simulink model "Z_3Dctrl"  (R2023a)
settings: Solver=ode1  StartTime=0.0  StopTime=inf  FixedStep=0.001  RelTol=1e-3  EnableMultiTasking=on
PostLoadFcn:
  | , if any(exist('dsrtsu_mdlpostloadfcn', 'file') ~= 0), dsrtsu_mdlpostloadfcn('Execute', bdroot); end,
InitFcn:
  | , if any(exist('rtifpga_mdlclblib', 'file') ~= 0), rtifpga_mdlclblib('Init', bdroot); end,
  | [b,a] = butter(6,0.6)
  | z0_default = 0.080001
  | fatness_default = 1
  | offset_default = 0
  | scale_default = 0
  | tic
model workspace (MAT data in the model file):
  Iters = 5
  N_coils = 6
  fatness_default = 1
  running = 0
  z0_default = 0.080001
undefined symbols (not defined in the file or in its folder): a, b, DiscIntNeverNeededParam
libraries: dspstat3 x7, simulink x5, commfilt2 x3, rti2004lib x3, rtilibm x1
(part 2 of 3)

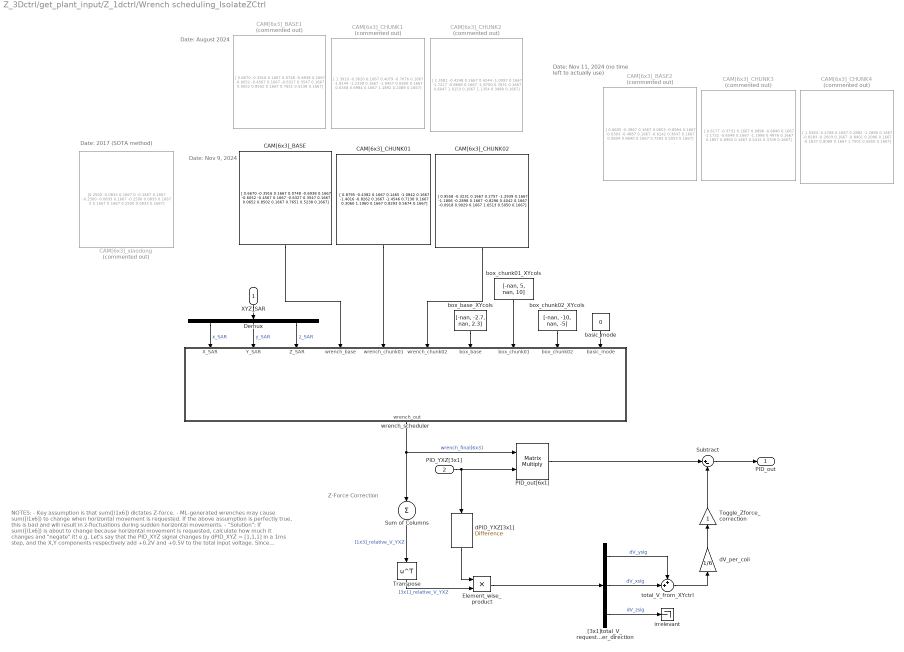
== system Z_3Dctrl/get_plant_input/Z_1dctrl/Wrench scheduling_IsolateZCtrl ==
  note: Date: August 2024
  note: Z-Force Correction
  note: NOTES:
      | - Key assumption is that sum([i1x6]) dictates Z-force.
      | - ML-generated wrenches may cause sum([i1x6]) to change when horizontal movement is requested. If the above assumption is perfectly true, this is bad and will result in z-fluctuations during sudden horizontal movements.
      | - "Solution": If sum([i1x6]) is about to change because horizontal movement is requested, calculate how much it changes and "negate" it!
      |
      | e.g. Let's say that the PID_XYZ signal changes by dPID_XYZ = [1,1,1] in a 1ms step, and the X,Y components respectively add +0.2V and +0.5V to the total input voltage.
      | Since sum(v[1x6]) is about to be +0.7V larger from horizontal motions alone (which is BAD since the sum, responsible for z-force, should be unaffected by horizontal motions), we "negate" this effect by subtracting (0.7V / 6 coils) = 0.11667V from EACH COIL in the final v[1x6] signal !
  note: Date: Nov 9, 2024
  note: Date: Nov 11, 2024
      | (no time left to actually use)
  note: Date: 2017 (SOTA method)
  XYZ_SAR : Inport
  PID_YXZ[3x1] : Inport  Port=2
  CAM[6x3]_BASE : Constant  Value=|
      | [    0.6670    -0.3916    0.1667
      |     0.0748    -0.6938    0.1667
      |    -0.6052   -0.4567    0.1667
      |    -0.6327   0.3547    0.1667
      |     0.0652   0.8502    0.1667
      |     0.7651   0.5238    0.1667]
  CAM[6x3]_BASE1 : Constant  Commented=on  Value=|
      | [    0.6670    -0.3916    0.1667
      |     0.0748    -0.6938    0.1667
      |    -0.6052   -0.4567    0.1667
      |    -0.6327   0.3547    0.1667
      |     0.0652   0.8502    0.1667
      |     0.7651   0.5238    0.1667]
  CAM[6x3]_BASE2 : Constant  Commented=on  Value=|
      | [    0.6605   -0.3967    0.1667
      |     0.0653   -0.8994    0.1667
      |    -0.6303   -0.4887    0.1667
      |    -0.6242    0.3647    0.1667
      |     0.0604    0.8640    0.1667
      |     0.7583    0.5053    0.1667]
  CAM[6x3]_CHUNK01 : Constant  Value=|
      | [    0.8795   -0.4382    0.1667
      |     0.1465   -1.0842    0.1667
      |    -1.4016   -0.8262    0.1667
      |    -1.4546    0.7130    0.1667
      |     0.3060    1.1960    0.1667
      |     0.8293    0.5674    0.1667]
  CAM[6x3]_CHUNK02 : Constant  Value=|
      | [   0.9558   -0.3231    0.1667
      |     0.2757   -1.2939    0.1667
      |    -1.1806   -0.2898    0.1667
      |    -0.8296    0.4042    0.1667
      |    -0.0918    0.9029    0.1667
      |     1.6513    0.5050    0.1667]
  CAM[6x3]_CHUNK1 : Constant  Commented=on  Value=|
      | [    1.3910    -0.3620    0.1667
      |     0.4079    -0.7676    0.1667
      |    -1.8144    -1.2338    0.1667
      |    -1.9457   0.6900    0.1667
      |     0.6358   0.6984    0.1667
      |     1.1892   0.2089    0.1667]
  CAM[6x3]_CHUNK2 : Constant  Commented=on  Value=|
      | [    1.3581    -0.4248    0.1667
      |     0.4244    -1.0097    0.1667
      |    -1.7217    -0.8668    0.1667
      |    -1.8700   0.7631    0.1667
      |     0.6047   1.0153    0.1667
      |     1.1354   0.3480    0.1667]
  CAM[6x3]_CHUNK3 : Constant  Commented=on  Value=|
      | [      0.6177   -0.3731    0.1667
      |     0.0896   -0.6840    0.1667
      |    -1.1732   -0.6548    0.1667
      |    -1.1996    0.4976    0.1667
      |     0.1857    0.6983    0.1667
      |     0.5415    0.3709    0.1667]
  CAM[6x3]_CHUNK4 : Constant  Commented=on  Value=|
      | [     1.0384   -0.4768    0.1667
      |     0.2882   -1.2890    0.1667
      |    -0.8283   -0.2003    0.1667
      |    -0.8401    0.2096    0.1667
      |    -0.1837    0.8089    0.1667
      |     1.7501    0.5650    0.1667]
  CAM[6x3]_xiaodong : Constant  Commented=on  Value=|
      | [0.2500    -0.0833    0.1667
      |          0    -0.1667    0.1667
      |    -0.2500    -0.0833    0.1667
      |    -0.2500   0.0833    0.1667
      |          0   0.1667    0.1667
      |     0.2500   0.0833    0.1667]
  Demux : Demux  Outputs=3
  Element_wise_product : Product
  PID_out[6x1] : Product  Multiplication=Matrix(*)
  Subtract : Sum  Inputs=|+-
  Sum of Columns : Sum  Inputs=+  CollapseMode=Specified dimension
  Toggle_Zforce_correction : Gain
  Transpose : Math  Operator=transpose
  "[3x1]total_V_requested_per_direction" : Demux  Outputs=3
  basic_mode : Constant  Value=0
  box_base_XYcols : Constant  Value=|
      | [-nan, -2.7,
      | nan, 2.3]
  box_chunk01_XYcols : Constant  Value=|
      | [-nan, 5,
      | nan, 10]
  box_chunk02_XYcols : Constant  Value=|
      | [-nan, -10,
      | nan, -5]
  dPID_YXZ[3x1] : simulink/Discrete/Difference  ICPrevInput=0.0  OutMin=[]  OutMax=[]  OutDataType=fixdt(1, 16)  OutScaling=2^-10  DoSatur=off
  dV_per_coil : Gain  Gain=1/6
  irrelevant : Terminator
  total_V_from_XYctrl : Sum  Inputs=++|
  wrench_scheduler : MATLAB Function  TreatAsAtomicUnit=on
  PID_out : Outport
  wires:
  CAM[6x3]_CHUNK02/1 -> wrench_scheduler/6(wrench_chunk02)
  box_chunk01_XYcols/1 -> wrench_scheduler/8(box_chunk01)
  basic_mode/1 -> wrench_scheduler/10(basic_mode)
  CAM[6x3]_BASE/1 -> wrench_scheduler/4(wrench_base)
  XYZ_SAR/1 -> Demux/1
  wrench_scheduler/1(wrench_out) -> Sum of Columns/1, PID_out[6x1]/1  "wrench_final[6x3]"
  Demux/3 -> wrench_scheduler/3(Z_SAR)  "z_SAR"
  box_base_XYcols/1 -> wrench_scheduler/7(box_base)
  CAM[6x3]_CHUNK01/1 -> wrench_scheduler/5(wrench_chunk01)
  Demux/2 -> wrench_scheduler/2(Y_SAR)  "y_SAR"
  Demux/1 -> wrench_scheduler/1(X_SAR)  "x_SAR"
  box_chunk02_XYcols/1 -> wrench_scheduler/9(box_chunk02)
  PID_out[6x1]/1 -> Subtract/1
  Sum of Columns/1 -> Transpose/1  "[1x3]_relative_V_YXZ"
  "[3x1]total_V_requested_per_direction"/1 -> total_V_from_XYctrl/1  "dV_ysig"
  "[3x1]total_V_requested_per_direction"/2 -> total_V_from_XYctrl/2  "dV_xsig"
  "[3x1]total_V_requested_per_direction"/3 -> irrelevant/1  "dV_zsig"
  PID_YXZ[3x1]/1 -> PID_out[6x1]/2, dPID_YXZ[3x1]/1
  Transpose/1 -> Element_wise_product/2  "[3x1]_relative_V_YXZ"
  Element_wise_product/1 -> "[3x1]total_V_requested_per_direction"/1
  dPID_YXZ[3x1]/1 -> Element_wise_product/1
  total_V_from_XYctrl/1 -> dV_per_coil/1
  dV_per_coil/1 -> Toggle_Zforce_correction/1
  Subtract/1 -> PID_out/1
  Toggle_Zforce_correction/1 -> Subtract/2

== system Z_3Dctrl/plant/Position Determination1/XY position Calculation ==
  note: !!MODIFIED!!
      | Before: "X_p, Y_p = Head2_read, Head3_read - radius_m".
      | After: "Head2_p, Head3_p = Head2_read, Head3_read + radius_m".
  note: Laser sensors output a voltage in [-10,10]V, proportional to the detected object's position in their 40mm FOV.
      | Conventions:
      | - Top of sensor (with large chamfer) is "up". Bottom of sensor is "down".
      | - "Upmost" measurement is -10V (-0.02m).
      | - "Downmost" measurement is +10V (+0.02m).
      | - Measurements go wonky if outer boundaries (+10V, -10V) are reached. For safety, do not let the magnet reach this range.
  Head II (Voltage) : Inport
  Head III (Voltage) : Inport  Port=2
  diameter_m : Inport  Port=3
  Mux : Mux  Inputs=2
  Sum : Sum  Inputs=|++
  Sum1 : Sum  Inputs=++|
  X_m : Fcn  Expr=(u(1)+u(2))*sin(pi/4)
  Y_m : Fcn  Expr=(u(1)-u(2))*sin(pi/4)
  diameter_to_radius : Gain  Gain=1/2
  volt_to_m : Gain  Gain=2/1000
  volt_to_m_2 : Gain  Gain=2/1000
  X_Position(m) : Outport
  Y_Position(m) : Outport  Port=2
  wires:
  Head III (Voltage)/1 -> volt_to_m_2/1
  Y_m/1 -> Y_Position(m)/1
  X_m/1 -> X_Position(m)/1
  Head II (Voltage)/1 -> volt_to_m/1
  Mux/1 -> Y_m/1, X_m/1
  Sum1/1 -> Mux/2  "Head3_p"
  volt_to_m_2/1 -> Sum1/2
  Sum/1 -> Mux/1  "Head2_p"
  diameter_to_radius/1 -> Sum1/1, Sum/2  "radius_m"
  volt_to_m/1 -> Sum/1
  diameter_m/1 -> diameter_to_radius/1

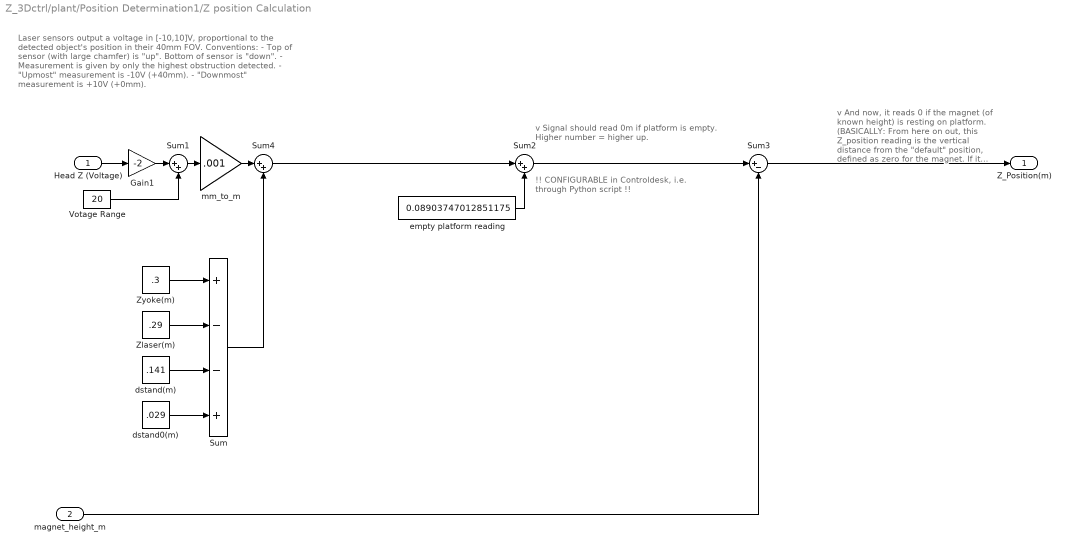
== system Z_3Dctrl/plant/Position Determination1/Z position Calculation ==
  note: Laser sensors output a voltage in [-10,10]V, proportional to the detected object's position in their 40mm FOV.
      | Conventions:
      | - Top of sensor (with large chamfer) is "up". Bottom of sensor is "down".
      | - Measurement is given by only the highest obstruction detected.
      | - "Upmost" measurement is -10V (+40mm).
      | - "Downmost" measurement is +10V (+0mm).
  note: v Signal should read 0m if platform is empty.
      | Higher number = higher up.
  note: v And now, it reads 0 if the magnet (of known height) is resting on platform.
      |
      | (BASICALLY: From here on out, this Z_position reading is the vertical distance from the "default" position, defined as zero for the magnet. If it reads something significantly different from 0, then double check the magnet height.)
  note: !! CONFIGURABLE in Controldesk, i.e. through Python script !!
  Head Z (Voltage) : Inport
  magnet_height_m : Inport  Port=2
  Gain1 : Gain  Gain=-2
  Sum : Sum  Inputs=+--+
  Sum1 : Sum  Inputs=|++
  Sum2 : Sum  Inputs=|++
  Sum3 : Sum  Inputs=|+-
  Sum4 : Sum  Inputs=|++
  Votage Range : Constant  Value=20
  Zlaser(m) : Constant  Value=.29
  Zyoke(m) : Constant  Value=.3
  dstand(m) : Constant  Value=.141
  dstand0(m) : Constant  Value=.029
  empty platform reading : Constant  Value=0.08903747012851175
  mm_to_m : Gain  Gain=.001
  Z_Position(m) : Outport
  wires:
  Sum2/1 -> Sum3/1
  Head Z (Voltage)/1 -> Gain1/1
  Sum/1 -> Sum4/2
  Sum1/1 -> mm_to_m/1
  Votage Range/1 -> Sum1/2
  Gain1/1 -> Sum1/1
  Zlaser(m)/1 -> Sum/2
  Zyoke(m)/1 -> Sum/1
  dstand(m)/1 -> Sum/3
  dstand0(m)/1 -> Sum/4
  magnet_height_m/1 -> Sum3/2
  Sum4/1 -> Sum2/1
  mm_to_m/1 -> Sum4/1
  empty platform reading/1 -> Sum2/2
  Sum3/1 -> Z_Position(m)/1

== system Z_3Dctrl/plant/Position Determination1/x filter ==
  u_raw : Inport
  10ms mean : Subsystem
  butter : DiscreteTransferFcn  Numerator=b  Denominator=a
  enable_butterworth : Constant
  enable_moving_mean : Constant
  switch_butter : Switch  Criteria=u2 > Threshold  SaturateOnIntegerOverflow=off  InputSameDT=off
  switch_movingmean : Switch  Criteria=u2 > Threshold  SaturateOnIntegerOverflow=off  InputSameDT=off
  u_filtered : Outport
  wires:
  enable_butterworth/1 -> switch_butter/2
  butter/1 -> switch_butter/1
  u_raw/1 -> switch_butter/3, butter/1
  enable_moving_mean/1 -> switch_movingmean/2
  switch_butter/1 -> 10ms mean/1(u), switch_movingmean/3
  10ms mean/1(movingmean(u)) -> switch_movingmean/1
  switch_movingmean/1 -> u_filtered/1

== system Z_3Dctrl/plant/Position Determination1/y filter ==
  u_raw : Inport
  10ms mean : Subsystem
  butter : DiscreteTransferFcn  Numerator=b  Denominator=a
  enable_butterworth : Constant
  enable_moving_mean : Constant
  switch_butter : Switch  Criteria=u2 > Threshold  SaturateOnIntegerOverflow=off  InputSameDT=off
  switch_movingmean : Switch  Criteria=u2 > Threshold  SaturateOnIntegerOverflow=off  InputSameDT=off
  u_filtered : Outport
  wires:
  enable_butterworth/1 -> switch_butter/2
  butter/1 -> switch_butter/1
  u_raw/1 -> switch_butter/3, butter/1
  enable_moving_mean/1 -> switch_movingmean/2
  switch_butter/1 -> 10ms mean/1(u), switch_movingmean/3
  10ms mean/1(movingmean(u)) -> switch_movingmean/1
  switch_movingmean/1 -> u_filtered/1

== system Z_3Dctrl/plant/Position Determination1/z filter SMOOTH ==
  u_raw : Inport
  10ms mean : Subsystem
  Terminator : Terminator
  Wn : Constant  Value=0.6
  butter2 : DiscreteTransferFcn  NumeratorSource=Input port  Numerator=b  DenominatorSource=Input port  Denominator=a  a0EqualsOne=on
      settings: InputPortMap=u0,p1,p3
  butterworth : MATLAB Function  TreatAsAtomicUnit=on
  enable_butterworth : Constant
  enable_moving_mean : Constant
  std_z : dspstat3/Moving Standard Deviation  Method=Sliding window  ForgettingFactorPort=off  SpecifyWindowLength=on  WindowLength=1000  OverlapLength=999  AllowArbitraryInputLength=off  ForgettingFactor=0.9  SimulateUsing=Code generation
  switch_butter : Switch  Criteria=u2 > Threshold  SaturateOnIntegerOverflow=off  InputSameDT=off
  switch_movingmean : Switch  Criteria=u2 > Threshold  SaturateOnIntegerOverflow=off  InputSameDT=off
  u_filtered : Outport
  wires:
  enable_butterworth/1 -> switch_butter/2
  u_raw/1 -> switch_butter/3, butter2/1
  enable_moving_mean/1 -> switch_movingmean/2
  switch_butter/1 -> 10ms mean/1(u), switch_movingmean/3
  10ms mean/1(movingmean(u)) -> switch_movingmean/1
  switch_movingmean/1 -> std_z/1, u_filtered/1
  Wn/1 -> butterworth/1(Wn)
  butterworth/2(aye) -> butter2/3
  butterworth/1(bee) -> butter2/2
  butter2/1 -> switch_butter/1
  std_z/1 -> Terminator/1

== system Z_3Dctrl/plant/output signal/output signal diagnostics ==
  H123_raw : Inport
  Discrete Transfer Fcn3 : DiscreteTransferFcn  Commented=on  NumeratorSource=Input port  Numerator=b  DenominatorSource=Input port  Denominator=a  a0EqualsOne=on
      settings: InputPortMap=u0,p1,p3
  Filtered signals : Demux  Commented=on  Outputs=3
  Mux : Mux  Inputs=3
  Raw signals : Demux  Outputs=3
  STDs : Subsystem  Commented=on
  Terminator1 : Terminator  Commented=on
  Terminator2 : Terminator  Commented=on
  Terminator3 : Terminator  Commented=on
  Wn : Constant  Commented=on  Value=0.9
  butterworth : MATLAB Function  Commented=on  TreatAsAtomicUnit=on
  center : Subsystem
  order : Constant  Commented=on  Value=6
  wires:
  Filtered signals/2 -> Terminator2/1  "HII_cen_fil"
  Filtered signals/3 -> Terminator3/1  "HIII_cen_fil"
  butterworth/1(bee) -> Discrete Transfer Fcn3/2
  butterworth/2(aye) -> Discrete Transfer Fcn3/3
  Discrete Transfer Fcn3/1 -> STDs/1(H123), Filtered signals/1
  order/1 -> butterworth/1(order)
  Wn/1 -> butterworth/2(Wn)
  H123_raw/1 -> center/1(u)
  Raw signals/1 -> Mux/1  "HZ_cen_raw"
  Raw signals/2 -> Mux/2  "HII_cen_raw"
  Raw signals/3 -> Mux/3  "HIII_cen_raw"
  Mux/1 -> Discrete Transfer Fcn3/1
  Filtered signals/1 -> Terminator1/1  "HZ_cen_fil"
  center/1(u_cen) -> Raw signals/1  "H123_cen_raw"

== system Z_3Dctrl/RTI Data/RTI Data Store/RTI Data Store/RTI Data Store ==
  RTI Data Store : Subsystem  mask(RTI_DATA_STORE){}
      mask help:
      | RTI Data Store Block. This block is used by RTI to store internal model dependent data. Deleting this block will result in data loss.
      |
      | NEVER DELETE, COPY, OR MODIFY THIS BLOCK!
      mask Help:
      | RTI Data Store Block. This block is used by RTI to store internal model dependent data. Deleting this block will result in data loss.
      | 
      | NEVER DELETE, COPY, OR MODIFY THIS BLOCK!
      mask Display: text(0.5, 0.5, ' ', 'HorizontalAlignment', 'center');

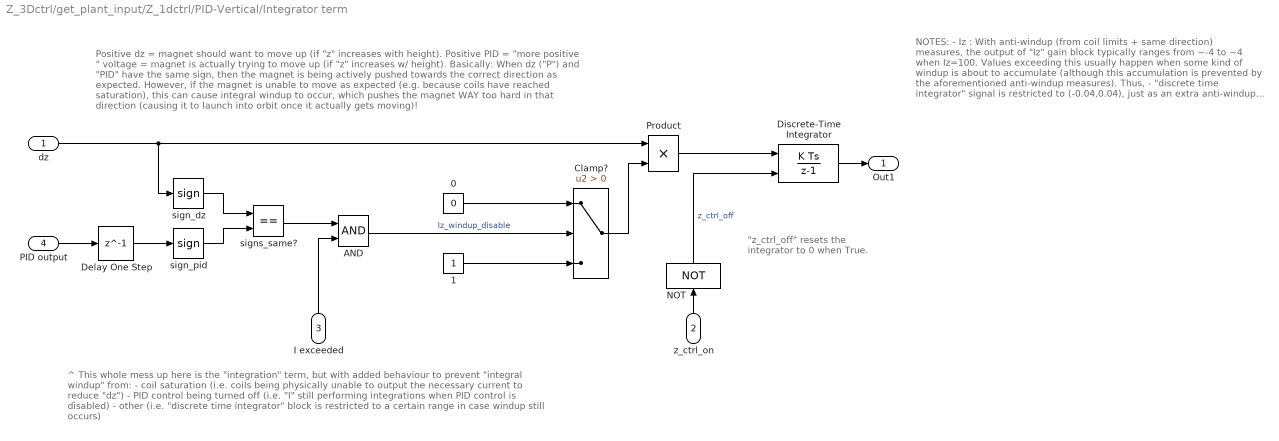
== system Z_3Dctrl/get_plant_input/Z_1dctrl/PID-Vertical/Integrator term ==
  note: "z_ctrl_off" resets the integrator to 0 when True.
  note: Positive dz = magnet should want to move up (if "z" increases with height).
      | Positive PID = "more positive " voltage = magnet is actually trying to move up (if "z" increases w/ height).
      |
      | Basically: When dz ("P") and "PID" have the same sign, then the magnet is being actively pushed towards the correct direction as expected. However, if the magnet is unable to move as expected (e.g. because coils have reached saturation), this can cause integral windup to occur, which pushes the magnet WAY too hard in that direction (causing it to launch into orbit once it actually gets moving)!
  note: NOTES:
      | - Iz : With anti-windup (from coil limits + same direction) measures, the output of "Iz" gain block typically ranges from ~-4 to ~4 when Iz=100. Values exceeding this usually happen when some kind of windup is about to accumulate (although this accumulation is prevented by the aforementioned anti-windup measures).
      | Thus,
      | - "discrete time integrator" signal is restricted to (-0.04,0.04), just as an extra anti-windup measure.
      | - Also, the integral resets while z-control is disabled.
  note: ^ This whole mess up here is the "integration" term, but with added behaviour to prevent "integral windup" from:
      | - coil saturation (i.e. coils being physically unable to output the necessary current to reduce "dz")
      | - PID control being turned off (i.e. "I" still performing integrations when PID control is disabled)
      | - other (i.e. "discrete time integrator" block is restricted to a certain range in case windup still occurs)
  dz : Inport
  z_ctrl_on : Inport  Port=2
  I exceeded : Inport  Port=3
  PID output : Inport  Port=4
  0 : Constant  Value=0
  1 : Constant
  AND : Logic  AllPortsSameDT=off  OutDataTypeStr=boolean
  Clamp? : Switch  Criteria=u2 > Threshold  SaturateOnIntegerOverflow=off  InputSameDT=off
  Delay One Step : Delay  DelayLength=1
  Discrete-Time Integrator : DiscreteIntegrator  ExternalReset=sampled level  SampleTime=-1  LimitOutput=on  UpperSaturationLimit=0.04  LowerSaturationLimit=-0.04  ICPrevOutput=DiscIntNeverNeededParam  ICPrevScaledInput=DiscIntNeverNeededParam
  NOT : Logic  Operator=NOT  AllPortsSameDT=off  OutDataTypeStr=boolean
  Product : Product
  sign_dz : Signum
  sign_pid : Signum
  signs_same? : RelationalOperator  Operator===  OutDataTypeStr=boolean  RndMeth=Simplest  InputSameDT=off
  Out1 : Outport
  wires:
  sign_dz/1 -> signs_same?/1
  AND/1 -> Clamp?/2  "Iz_windup_disable"
  signs_same?/1 -> AND/1
  sign_pid/1 -> signs_same?/2
  1/1 -> Clamp?/3
  NOT/1 -> Discrete-Time Integrator/2  "z_ctrl_off"
  0/1 -> Clamp?/1
  Product/1 -> Discrete-Time Integrator/1
  dz/1 -> sign_dz/1, Product/1
  Clamp?/1 -> Product/2
  PID output/1 -> Delay One Step/1
  Discrete-Time Integrator/1 -> Out1/1
  z_ctrl_on/1 -> NOT/1
  I exceeded/1 -> AND/2
  Delay One Step/1 -> sign_pid/1

== system Z_3Dctrl/get_plant_input/Z_1dctrl/PID-Vertical/PID Gain scheduler ==
  Zd : Inport
  dz : Inport  Port=2
  Dz : Constant  Value=nan
  Iz : Constant  Value=nan
  PID selector : MATLAB Function  TreatAsAtomicUnit=on
  Pz : Constant  Value=nan
  "[Pz, Iz, Dz_outer, Dz_inner, z] array" : Constant  Value=[400 2000 3200 3200 0.002; 310 350 5500 4000 0.005]
  dz_inner_threshold_mm : Constant  Value=0.1
  dz_outer_threshold_mm : Constant  Value=0.25
  PID_gains : Outport
  wires:
  Zd/1 -> PID selector/1(Zd)
  Iz/1 -> PID selector/7(I_override)
  Dz/1 -> PID selector/8(D_override)
  dz/1 -> PID selector/2(dz)
  dz_outer_threshold_mm/1 -> PID selector/5(dz_outer_threshold)
  "[Pz, Iz, Dz_outer, Dz_inner, z] array"/1 -> PID selector/3(PIDDz_save)
  Pz/1 -> PID selector/6(P_override)
  dz_inner_threshold_mm/1 -> PID selector/4(dz_inner_threshold)
  PID selector/1(PID_out) -> PID_gains/1

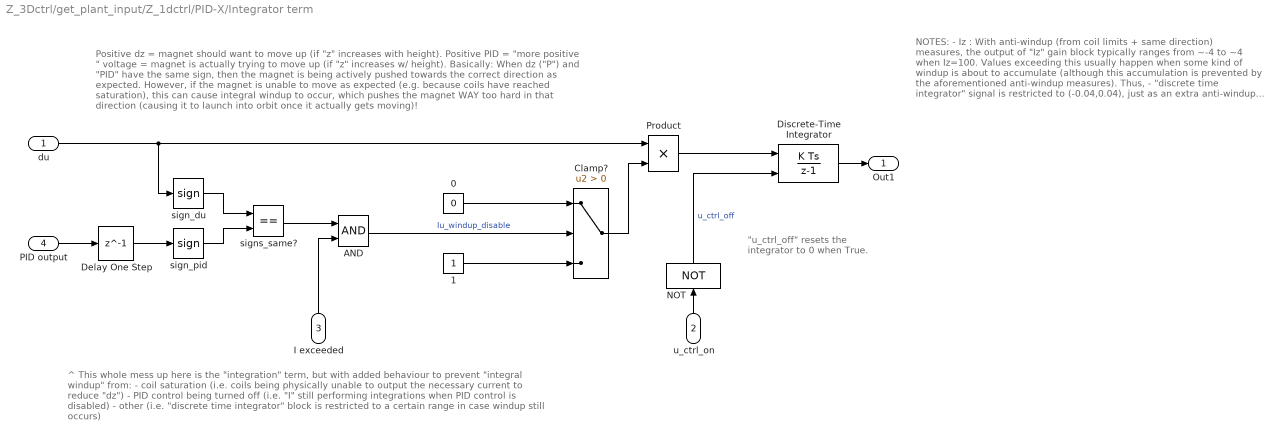
== system Z_3Dctrl/get_plant_input/Z_1dctrl/PID-X/Integrator term ==
  note: "u_ctrl_off" resets the integrator to 0 when True.
  note: Positive dz = magnet should want to move up (if "z" increases with height).
      | Positive PID = "more positive " voltage = magnet is actually trying to move up (if "z" increases w/ height).
      |
      | Basically: When dz ("P") and "PID" have the same sign, then the magnet is being actively pushed towards the correct direction as expected. However, if the magnet is unable to move as expected (e.g. because coils have reached saturation), this can cause integral windup to occur, which pushes the magnet WAY too hard in that direction (causing it to launch into orbit once it actually gets moving)!
  note: NOTES:
      | - Iz : With anti-windup (from coil limits + same direction) measures, the output of "Iz" gain block typically ranges from ~-4 to ~4 when Iz=100. Values exceeding this usually happen when some kind of windup is about to accumulate (although this accumulation is prevented by the aforementioned anti-windup measures).
      | Thus,
      | - "discrete time integrator" signal is restricted to (-0.04,0.04), just as an extra anti-windup measure.
      | - Also, the integral resets while z-control is disabled.
  note: ^ This whole mess up here is the "integration" term, but with added behaviour to prevent "integral windup" from:
      | - coil saturation (i.e. coils being physically unable to output the necessary current to reduce "dz")
      | - PID control being turned off (i.e. "I" still performing integrations when PID control is disabled)
      | - other (i.e. "discrete time integrator" block is restricted to a certain range in case windup still occurs)
  du : Inport
  u_ctrl_on : Inport  Port=2
  I exceeded : Inport  Port=3
  PID output : Inport  Port=4
  0 : Constant  Value=0
  1 : Constant
  AND : Logic  AllPortsSameDT=off  OutDataTypeStr=boolean
  Clamp? : Switch  Criteria=u2 > Threshold  SaturateOnIntegerOverflow=off  InputSameDT=off
  Delay One Step : Delay  DelayLength=1
  Discrete-Time Integrator : DiscreteIntegrator  ExternalReset=sampled level  SampleTime=-1  LimitOutput=on  UpperSaturationLimit=0.04  LowerSaturationLimit=-0.04  ICPrevOutput=DiscIntNeverNeededParam  ICPrevScaledInput=DiscIntNeverNeededParam
  NOT : Logic  Operator=NOT  AllPortsSameDT=off  OutDataTypeStr=boolean
  Product : Product
  sign_du : Signum
  sign_pid : Signum
  signs_same? : RelationalOperator  Operator===  OutDataTypeStr=boolean  RndMeth=Simplest  InputSameDT=off
  Out1 : Outport
  wires:
  sign_du/1 -> signs_same?/1
  AND/1 -> Clamp?/2  "Iu_windup_disable"
  signs_same?/1 -> AND/1
  sign_pid/1 -> signs_same?/2
  1/1 -> Clamp?/3
  NOT/1 -> Discrete-Time Integrator/2  "u_ctrl_off"
  0/1 -> Clamp?/1
  Product/1 -> Discrete-Time Integrator/1
  du/1 -> sign_du/1, Product/1
  Clamp?/1 -> Product/2
  PID output/1 -> Delay One Step/1
  Discrete-Time Integrator/1 -> Out1/1
  u_ctrl_on/1 -> NOT/1
  I exceeded/1 -> AND/2
  Delay One Step/1 -> sign_pid/1

== system Z_3Dctrl/get_plant_input/Z_1dctrl/PID-X/PID Gain scheduler ==
  Ud : Inport
  du : Inport  Port=2
  Du : Constant  Value=1500
  Iu : Constant  Value=70
  Mux : Mux  Inputs=3
  PID selector : MATLAB Function  Commented=on  TreatAsAtomicUnit=on
  Pu : Constant  Value=20
  Terminator : Terminator  Commented=on
  Terminator1 : Terminator
  Terminator2 : Terminator
  "[Pu, Iu, Du_outer, Du_inner, z] array" : Constant  Commented=on  Value=[400 2000 3200 3200 0.002; 310 350 5500 4000 0.005]
  du_inner_threshold_mm : Constant  Commented=on  Value=0.1
  du_outer_threshold_mm : Constant  Commented=on  Value=0.25
  PID_gains : Outport
  wires:
  Ud/1 -> Terminator1/1
  Iu/1 -> Mux/2
  Du/1 -> Mux/3
  du/1 -> Terminator2/1
  du_outer_threshold_mm/1 -> PID selector/5(du_outer_threshold)
  "[Pu, Iu, Du_outer, Du_inner, z] array"/1 -> PID selector/3(PIDDu_save)
  Pu/1 -> Mux/1
  du_inner_threshold_mm/1 -> PID selector/4(du_inner_threshold)
  PID selector/1(PID_out) -> Terminator/1
  Mux/1 -> PID_gains/1

== system Z_3Dctrl/get_plant_input/Z_1dctrl/PID-Y/Integrator term ==
  note: "u_ctrl_off" resets the integrator to 0 when True.
  note: Positive dz = magnet should want to move up (if "z" increases with height).
      | Positive PID = "more positive " voltage = magnet is actually trying to move up (if "z" increases w/ height).
      |
      | Basically: When dz ("P") and "PID" have the same sign, then the magnet is being actively pushed towards the correct direction as expected. However, if the magnet is unable to move as expected (e.g. because coils have reached saturation), this can cause integral windup to occur, which pushes the magnet WAY too hard in that direction (causing it to launch into orbit once it actually gets moving)!
  note: NOTES:
      | - Iz : With anti-windup (from coil limits + same direction) measures, the output of "Iz" gain block typically ranges from ~-4 to ~4 when Iz=100. Values exceeding this usually happen when some kind of windup is about to accumulate (although this accumulation is prevented by the aforementioned anti-windup measures).
      | Thus,
      | - "discrete time integrator" signal is restricted to (-0.04,0.04), just as an extra anti-windup measure.
      | - Also, the integral resets while z-control is disabled.
  note: ^ This whole mess up here is the "integration" term, but with added behaviour to prevent "integral windup" from:
      | - coil saturation (i.e. coils being physically unable to output the necessary current to reduce "dz")
      | - PID control being turned off (i.e. "I" still performing integrations when PID control is disabled)
      | - other (i.e. "discrete time integrator" block is restricted to a certain range in case windup still occurs)
  du : Inport
  u_ctrl_on : Inport  Port=2
  I exceeded : Inport  Port=3
  PID output : Inport  Port=4
  0 : Constant  Value=0
  1 : Constant
  AND : Logic  AllPortsSameDT=off  OutDataTypeStr=boolean
  Clamp? : Switch  Criteria=u2 > Threshold  SaturateOnIntegerOverflow=off  InputSameDT=off
  Delay One Step : Delay  DelayLength=1
  Discrete-Time Integrator : DiscreteIntegrator  ExternalReset=sampled level  SampleTime=-1  LimitOutput=on  UpperSaturationLimit=0.04  LowerSaturationLimit=-0.04  ICPrevOutput=DiscIntNeverNeededParam  ICPrevScaledInput=DiscIntNeverNeededParam
  NOT : Logic  Operator=NOT  AllPortsSameDT=off  OutDataTypeStr=boolean
  Product : Product
  sign_du : Signum
  sign_pid : Signum
  signs_same? : RelationalOperator  Operator===  OutDataTypeStr=boolean  RndMeth=Simplest  InputSameDT=off
  Out1 : Outport
  wires:
  sign_du/1 -> signs_same?/1
  AND/1 -> Clamp?/2  "Iu_windup_disable"
  signs_same?/1 -> AND/1
  sign_pid/1 -> signs_same?/2
  1/1 -> Clamp?/3
  NOT/1 -> Discrete-Time Integrator/2  "u_ctrl_off"
  0/1 -> Clamp?/1
  Product/1 -> Discrete-Time Integrator/1
  du/1 -> sign_du/1, Product/1
  Clamp?/1 -> Product/2
  PID output/1 -> Delay One Step/1
  Discrete-Time Integrator/1 -> Out1/1
  u_ctrl_on/1 -> NOT/1
  I exceeded/1 -> AND/2
  Delay One Step/1 -> sign_pid/1

== system Z_3Dctrl/get_plant_input/Z_1dctrl/PID-Y/PID Gain scheduler ==
  Ud : Inport
  du : Inport  Port=2
  Du : Constant  Value=1500
  Iu : Constant  Value=70
  Mux : Mux  Inputs=3
  PID selector : MATLAB Function  Commented=on  TreatAsAtomicUnit=on
  Pu : Constant  Value=20
  Terminator : Terminator  Commented=on
  Terminator1 : Terminator
  Terminator2 : Terminator
  "[Pu, Iu, Du_outer, Du_inner, z] array" : Constant  Commented=on  Value=[400 2000 3200 3200 0.002; 310 350 5500 4000 0.005]
  du_inner_threshold_mm : Constant  Commented=on  Value=0.1
  du_outer_threshold_mm : Constant  Commented=on  Value=0.25
  PID_gains : Outport
  wires:
  Ud/1 -> Terminator1/1
  Iu/1 -> Mux/2, PID selector/7(I_override)
  Du/1 -> Mux/3, PID selector/8(D_override)
  du/1 -> Terminator2/1
  du_outer_threshold_mm/1 -> PID selector/5(du_outer_threshold)
  "[Pu, Iu, Du_outer, Du_inner, z] array"/1 -> PID selector/3(PIDDu_save)
  Pu/1 -> Mux/1, PID selector/6(P_override)
  du_inner_threshold_mm/1 -> PID selector/4(du_inner_threshold)
  PID selector/1(PID_out) -> Terminator/1
  Mux/1 -> PID_gains/1

== system Z_3Dctrl/plant/Position Determination1/x filter/10ms mean ==
  note: NOTE: Sensor readings fluctuate over a peak-to-peak amplitude of about 4.5e-5 m, over a period of almost exactly 10ms.
      |
      | 08/14/23: See how it improves if I only consider the mean signal over 10ms!
  u : Inport
  ave signal : Product  Inputs=*/
  integration window (samples) : Constant  Value=10
  sum of signal over short time : commfilt2/Windowed Integrator  integperiod=10  InputProcessing=Columns as channels (frame based)  roundingMode=Floor  overflowMode=off  coeffDataTypeStr=Inherit: Same word length as input  coeffMin=[]  coeffMax=[]  coeffLastDataTypeStr=Inherit: Same word length as input  accumDataTypeStr=Inherit: Same as product output  accumLastDataTypeStr=Inherit: Same as product output  outputDataTypeStr=Inherit: Same as accumulator  outputMin=[]  outputMax=[]  outputLastDataTypeStr=Inherit: Same as accumulator
  movingmean(u) : Outport
  wires:
  sum of signal over short time/1 -> ave signal/1
  u/1 -> sum of signal over short time/1
  integration window (samples)/1 -> ave signal/2
  ave signal/1 -> movingmean(u)/1

== system Z_3Dctrl/plant/Position Determination1/y filter/10ms mean ==
  note: NOTE: Sensor readings fluctuate over a peak-to-peak amplitude of about 4.5e-5 m, over a period of almost exactly 10ms.
      |
      | 08/14/23: See how it improves if I only consider the mean signal over 10ms!
  u : Inport
  ave signal : Product  Inputs=*/
  integration window (samples) : Constant  Value=10
  sum of signal over short time : commfilt2/Windowed Integrator  integperiod=10  InputProcessing=Columns as channels (frame based)  roundingMode=Floor  overflowMode=off  coeffDataTypeStr=Inherit: Same word length as input  coeffMin=[]  coeffMax=[]  coeffLastDataTypeStr=Inherit: Same word length as input  accumDataTypeStr=Inherit: Same as product output  accumLastDataTypeStr=Inherit: Same as product output  outputDataTypeStr=Inherit: Same as accumulator  outputMin=[]  outputMax=[]  outputLastDataTypeStr=Inherit: Same as accumulator
  movingmean(u) : Outport
  wires:
  sum of signal over short time/1 -> ave signal/1
  u/1 -> sum of signal over short time/1
  integration window (samples)/1 -> ave signal/2
  ave signal/1 -> movingmean(u)/1

== system Z_3Dctrl/plant/Position Determination1/z filter SMOOTH/10ms mean ==
  note: NOTE: Sensor readings fluctuate over a peak-to-peak amplitude of about 4.5e-5 m, over a period of almost exactly 10ms.
      |
      | 08/14/23: See how it improves if I only consider the mean signal over 10ms!
  u : Inport
  ave signal : Product  Inputs=*/
  integration window (samples) : Constant  Value=10
  sum of signal over short time : commfilt2/Windowed Integrator  integperiod=10  InputProcessing=Columns as channels (frame based)  roundingMode=Floor  overflowMode=off  coeffDataTypeStr=Inherit: Same word length as input  coeffMin=[]  coeffMax=[]  coeffLastDataTypeStr=Inherit: Same word length as input  accumDataTypeStr=Inherit: Same as product output  accumLastDataTypeStr=Inherit: Same as product output  outputDataTypeStr=Inherit: Same as accumulator  outputMin=[]  outputMax=[]  outputLastDataTypeStr=Inherit: Same as accumulator
  movingmean(u) : Outport
  wires:
  sum of signal over short time/1 -> ave signal/1
  u/1 -> sum of signal over short time/1
  integration window (samples)/1 -> ave signal/2
  ave signal/1 -> movingmean(u)/1

== system Z_3Dctrl/plant/output signal/output signal diagnostics/STDs ==
  H123 : Inport
  Demux : Demux  Outputs=3
  Moving Standard Deviation : dspstat3/Moving Standard Deviation  Method=Sliding window  ForgettingFactorPort=off  SpecifyWindowLength=on  WindowLength=3000  OverlapLength=2999  AllowArbitraryInputLength=off  ForgettingFactor=0.9  SimulateUsing=Code generation
  Moving Standard Deviation1 : dspstat3/Moving Standard Deviation  Method=Sliding window  ForgettingFactorPort=off  SpecifyWindowLength=on  WindowLength=3000  OverlapLength=2999  AllowArbitraryInputLength=off  ForgettingFactor=0.9  SimulateUsing=Code generation
  Moving Standard Deviation2 : dspstat3/Moving Standard Deviation  Method=Sliding window  ForgettingFactorPort=off  SpecifyWindowLength=on  WindowLength=3000  OverlapLength=2999  AllowArbitraryInputLength=off  ForgettingFactor=0.9  SimulateUsing=Code generation
  Terminator : Terminator
  Terminator1 : Terminator
  Terminator2 : Terminator
  wires:
  H123/1 -> Demux/1
  Demux/1 -> Moving Standard Deviation/1
  Demux/2 -> Moving Standard Deviation1/1
  Demux/3 -> Moving Standard Deviation2/1
  Moving Standard Deviation/1 -> Terminator/1  "std_HZ"
  Moving Standard Deviation1/1 -> Terminator1/1  "std_HII"
  Moving Standard Deviation2/1 -> Terminator2/1  "std_HIII"

== system Z_3Dctrl/plant/output signal/output signal diagnostics/center ==
  u : Inport
  Demux : Demux  Outputs=3
  Moving Average : dspstat3/Moving Average  Method=Sliding window  ForgettingFactorPort=off  SpecifyWindowLength=on  WindowLength=3000  OverlapLength=2999  AllowArbitraryInputLength=off  ForgettingFactor=0.9  SimulateUsing=Code generation
  Moving Average1 : dspstat3/Moving Average  Method=Sliding window  ForgettingFactorPort=off  SpecifyWindowLength=on  WindowLength=3000  OverlapLength=2999  AllowArbitraryInputLength=off  ForgettingFactor=0.9  SimulateUsing=Code generation
  Moving Average2 : dspstat3/Moving Average  Method=Sliding window  ForgettingFactorPort=off  SpecifyWindowLength=on  WindowLength=3000  OverlapLength=2999  AllowArbitraryInputLength=off  ForgettingFactor=0.9  SimulateUsing=Code generation
  Mux : Mux  Inputs=3
  Sum : Sum  Inputs=|+-
  Sum1 : Sum  Inputs=|+-
  Sum2 : Sum  Inputs=|+-
  u_cen : Outport
  wires:
  u/1 -> Demux/1
  Moving Average/1 -> Sum/2
  Demux/1 -> Sum/1, Moving Average/1
  Moving Average1/1 -> Sum1/2
  Demux/2 -> Moving Average1/1, Sum1/1
  Moving Average2/1 -> Sum2/2
  Demux/3 -> Moving Average2/1, Sum2/1
  Sum1/1 -> Mux/2
  Sum/1 -> Mux/1
  Sum2/1 -> Mux/3
  Mux/1 -> u_cen/1

== system Z_3Dctrl/RTI Data/RTI Data Store/RTI Data Store/RTI Data Store/RTI Data Store ==

== matlab function Z_3Dctrl/plant/output signal/output signal diagnostics/butterworth ==
  data: order input; bee output; Wn input; aye output
function [bee,aye] = butterwort(order,Wn)
% order = order of lowpass Butterworth filter
% Wn = NORMALIZED cutoff frequency
%    = fc/(fs/2), where fc = cutoff frequency (Hz),
%                       fs = sample frequency (Hz) (1000 for our system)
%    = ratio between cutoff frequency and HALF of sample frequency!

% Ignore the order actually lmao
order = 2;
[bee,aye] = butter(order,Wn);

== matlab function Z_3Dctrl/plant/Position Determination1/z filter SMOOTH/butterworth ==
  data: bee output; Wn input; aye output
function [bee,aye] = butterwort(Wn)
% order = order of lowpass Butterworth filter
% Wn = NORMALIZED cutoff frequency
%    = fc/(fs/2), where fc = cutoff frequency (Hz),
%                       fs = sample frequency (Hz) (1000 for our system)
%    = ratio between cutoff frequency and HALF of sample frequency!

% Ignore the order actually lmao
order = 6;
[bee,aye] = butter(order,Wn);

== matlab function Z_3Dctrl/get_plant_input/Z_1dctrl/Wrench scheduling_IsolateZCtrl/wrench_scheduler ==
  data: X_SAR input; Y_SAR input; Z_SAR input; wrench_out output; wrench_base input; wrench_chunk01 input; wrench_chunk02 input; box_base input; box_chunk01 input; box_chunk02 input; basic_mode input
function wrench_out = fcn(X_SAR,Y_SAR,Z_SAR,wrench_base,wrench_chunk01,wrench_chunk02,box_base,box_chunk01,box_chunk02,basic_mode)
% Smoothly chooses the wrench matrix to use based on how far away the
% magnet is from the "BASE" wrench's bounding box (on which it was
% trained).
% (08-23-24) For the time being, high Y values mean using Chunk01's wrench,
% and low Y values mean using Chunk02's wrench.

% Read recorded PID gains
x = X_SAR(1);
y = Y_SAR(1);
z = Z_SAR(1);

% Ps = PIDDz_save(:,1);
% Is = PIDDz_save(:,2);
% Douts = PIDDz_save(:,3);
% Dins = PIDDz_save(:,4);
% Zs = PIDDz_save(:,5);
% [~,lowest_index] = min(Zs);
% [~,highest_index] = max(Zs);

% Box range
box_base_xmin = box_base(1,1)/1000;
box_base_xmax = box_base(2,1)/1000;
box_base_ymin = box_base(1,2)/1000;
box_base_ymax = box_base(2,2)/1000;

% Chunk01 range
box_chunk01_xmin = box_chunk01(1,1)/1000;
box_chunk01_xmax = box_chunk01(2,1)/1000;
box_chunk01_ymin = box_chunk01(1,2)/1000;
box_chunk01_ymax = box_chunk01(2,2)/1000;
box_chunk01_ymean = (box_chunk01_ymin+box_chunk01_ymax)/2;
% Chunk02 range
box_chunk02_xmin = box_chunk02(1,1)/1000;
box_chunk02_xmax = box_chunk02(2,1)/1000;
box_chunk02_ymin = box_chunk02(1,2)/1000;
box_chunk02_ymax = box_chunk02(2,2)/1000;
box_chunk02_ymean = (box_chunk02_ymin+box_chunk02_ymax)/2;


% Interpolate if necessary!
if basic_mode==2
    xiaodong_wrench =  [0.2500    -0.0833    0.1667
                             0    -0.1667    0.1667
                       -0.2500    -0.0833    0.1667
                       -0.2500     0.0833    0.1667
                             0     0.1667    0.1667
                        0.2500     0.0833    0.1667];
    xiaodong_wrench_XY_scaler = [2.6    0   0
                                   0  2.6   0
                                   0    0   1];
    wrench = xiaodong_wrench * xiaodong_wrench_XY_scaler;
elseif (y <= box_base_ymax && y >= box_base_ymin) || basic_mode==1
    % disp("Inside base chunk!")
    wrench = wrench_base;

elseif y >= box_base_ymax
    % disp("Start using chunk01!")
    wrench_scale = min(1,(y - box_base_ymax)/(box_chunk01_ymean-box_base_ymax));
    wrench = wrench_base*(1-wrench_scale) + wrench_chunk01*(wrench_scale);
else
    % disp("Start using chunk02!")
    wrench_scale = min(1,(box_base_ymin - y)/(box_base_ymin - box_chunk02_ymean));
    wrench = wrench_base*(1-wrench_scale) + wrench_chunk02*(wrench_scale);
end

% Apply scaled wrench!
wrench_out = wrench;

== matlab function Z_3Dctrl/Input parameters/parametric_path_tracer ==
  data: t input; XYZ_d output; mode input; enable_3D input
function XYZ_d = parametric_path_tracer(t,mode,enable_3D)

% Parameters
ymax = 0.006;       % Max y-distance from origin
xmax = 0.002;       % Max x-distance from origin
dz = 0.0015;     % Deviation in height from start
z_init = 0.002;    % Starting z-value

tmax = 30;      % Assumed duration of path tracing
% ^ DEFINE: tmax (in seconds) is where measurement ENDS; helix dimensions
% are decided based on this!


switch mode
    case 0
        % OVAL
        freq = 1/30;     % full rotations per second (helix only)
        % Parametric equations
        x = (xmax ) .* cos(2*pi*freq * t);
        y = (ymax ) .* sin(2*pi*freq * t);
        z = z_init + enable_3D*(dz) * sin(2*pi*freq * t);
    case 1
        % HELIX (TORNADO)
        freq = 0.08;     % full rotations per second (helix only)
        % Parametric equations
        x = (xmax * t / tmax) .* cos(2*pi*freq * t);
        y = (ymax * t / tmax) .* sin(2*pi*freq * t);
        z = z_init + (dz) * t / tmax * enable_3D;
    case 2
        % HELIX (DRILL)
        freq = 0.2;     % full rotations per second (helix only)
        % Parametric equations
        x = (xmax * t / tmax) .* cos(2*pi*freq * t);
        y = -ymax + (2*ymax * t / tmax);
        z = z_init + (dz) * t / tmax  .* sin(2*pi*freq * t) * enable_3D;
    case 3
        % FIGURE 8
        freq = 1/30;     % full rotations per second (helix only)
        % Parametric equations
        x = (xmax ) .* sin(2*pi*freq * 2*t);
        y = (ymax ) .* sin(2*pi*freq * t);
        z = z_init + enable_3D * (dz) * sin(2*pi*freq * t);
    case 4
        % RECTANGLE
        % Parameters
        w = 2*xmax;    % Width of the rectangle
        h = 2*ymax;    % Height of the rectangle
        k = dz / ymax;    % Tilt factor for the z-direction (rise/run)
       
        
        % Define each segment of the rectangle based on the proportional value of t
        segment = t / (tmax / 4);  % Scale t to 4 segments
        
        % First edge (right vertical; start at top right)
        if (segment < 1)
            x = w / 2;
            y = h / 2 - segment * h;
            z = enable_3D *k * y + z_init;
        
        % Second edge (bottom horizontal)
        elseif (segment >= 1) && (segment < 2)
            x = w / 2 - mod(segment,1)*w;
            y = -h / 2;
            z = enable_3D *k * y  + z_init;
        
        % Third edge (left vertical)
        elseif (segment >= 2) && (segment < 3)
            x = -w / 2;
            y = -h / 2 + mod(segment,1) * h;
            z = enable_3D *k * y + z_init;
        
        % Fourth edge (top horizontal)
        elseif (segment >= 3) && (segment < 4)
            x = -w / 2 + mod(segment,1)*w;
            y = h / 2;
            z = enable_3D *k * y + z_init;
        else
            x = w/2;
            y = h/2;
            z = enable_3D *k * y + z_init;
        end

    otherwise
        x = 0;
        y = 0;
        z = 0;
end

XYZ_d = [x; y; z];

== matlab function Z_3Dctrl/Input parameters/Magnet Specs/Magnet Physical Specs ==
  data: unit_mode input; diameter input; height input; diameter_m output; height_m output; mass_g output; B_r output; mass input; magnet_remanence_t input; errorflag output
function [diameter_m,height_m,mass_g,B_r,errorflag]= mag_specs(unit_mode,diameter,height,mass,magnet_remanence_t)
% User can specify parameters for cylindrical magnets: diameter, height 
% (units: "in" or "cm" or "mm" or "m"), mass, and either remanent B-field
% (in T or G) or magnetic dipole moment (in N*m/T, aka A*m^2).
% TO IMPLEMENT: Ring magnets!

errorflag = 0;

%%% DIMENSIONS %%%
% Dimensions, in m
% NOTE: Unit modes are:
% 1 - m
% 2 - cm
% 3 - mm
% 4 - in
if unit_mode==1
    units_to_m = 1;
elseif unit_mode==2
    units_to_m = 0.01;
elseif unit_mode==3
    units_to_m = 0.001;
elseif unit_mode==4
    units_to_m = 0.0254;
else
    % (TEMP?) Assume that the user wants metres
    units_to_m = 1;
end

% Dimensions
% if isnan(diameter)
%     diameter = diameter_detect;
% end
% if isnan(diameter_detect)
%     diameter_detect = diameter;
% end
% if isnan(height)
%     height = height_detect;
% end
% if isnan(height_detect)
%     height_detect = height;
% end
diameter_m = diameter * units_to_m;
height_m = height * units_to_m;
mass_g = mass;

%%% MAG FIELD STUFF %%%
% Mag field info (Br in Gauss or T)
if magnet_remanence_t > 1000
    % Assumes a remanence field value based on the material, in Gauss.
    % For example, an N52 magnet has 14800G, and Xiaodong's now-battered
    % magnet has 12900G.
    B_r = magnet_remanence_t / 10000;
else
    % Assumes a remanence field value based on the material, in T.
    % For example, an N52 magnet has 1.48T, and Xiaodong's now-battered
    % magnet has 1.29T.
    B_r = magnet_remanence_t / 1;
end

% (!!!!) CREATE CHART FOR CONVERSION FROM Nxx FORMAT TO REMANENCE IN T

% K&J SPECS:
%     % Assumes a grade was inputted as a string-- N52, N42, etc!
%     if lower(magfield_grade_t)=="n52"
%         B_r = 1.48;
%     elseif lower(magfield_grade_t)=="n50"
%         B_r = 1.45;
%     elseif lower(magfield_grade_t)=="n48"
%         B_r = 1.42;
%     elseif lower(magfield_grade_t)=="n45"
%         B_r = 1.35;
%     elseif lower(magfield_grade_t)=="n42"
%         B_r = 1.32;
%     elseif lower(magfield_grade_t)=="n40"
%         B_r = 1.29;
%     elseif lower(magfield_grade_t)=="n35"
%         B_r = 1.21;
%     else
%         % SHOULD NEVER HAPPEN
%         B_r = 1.48;
%         errorflag = 1;
%     end
% APPLIEDMAGNETS SPECS:
%     % Assumes a grade was inputted as a string-- N52, N42, etc!
%     if lower(magfield_grade_t)=="n52"
%         B_r = 1.48;
%     elseif lower(magfield_grade_t)=="n50"
%         B_r = 1.45;
%     elseif lower(magfield_grade_t)=="n48"
%         B_r = 1.42;
%     elseif lower(magfield_grade_t)=="n45"
%         B_r = 1.38 (rarely 1.35);
%     elseif lower(magfield_grade_t)=="n42"
%         B_r = 1.32;
%     elseif lower(magfield_grade_t)=="n40"
%         B_r = 1.29;
%     else
%         % SHOULD NEVER HAPPEN
%         B_r = 1.48;
%         errorflag = 1;
%     end
% 
% 
%

== matlab function Z_3Dctrl/get_plant_input/Z_1dctrl/PID-X/PID Gain scheduler/PID selector ==
  data: Ud input; du input; PIDDu_save input; du_inner_threshold input; du_outer_threshold input; PID_out output; P_override input; I_override input; D_override input
function PID_out = fcn(Ud,du,PIDDu_save,du_inner_threshold, du_outer_threshold, P_override,I_override,D_override)
% Interpolates for PID gains based on target Ud, using PID gains that were
% manually tuned at various target "Z" heights (with D gain being split into
% "near target height" and "far from target height" values, to allow for
% strong D contribution without risking destabilization near convergence).
% The "D" gain is then chosen between these aforementioned values based on
% how near/far the magnet is to Zd.

% Read recorded PID gains
Zq = Ud;

Ps = PIDDu_save(:,1);
Is = PIDDu_save(:,2);
Douts = PIDDu_save(:,3);
Dins = PIDDu_save(:,4);
Zs = PIDDu_save(:,5);
[~,lowest_index] = min(Zs);
[~,highest_index] = max(Zs);


% Interpolate if necessary!
if Ud <= Zs(lowest_index)
    % disp("Below 2mm!")
    P_final = Ps(lowest_index);
    I_final = Is(lowest_index);
    Dout_final = Douts(lowest_index);
    Din_final  = Dins(lowest_index);
elseif Ud >= Zs(highest_index)
    % disp("Above 5mm!")
    P_final = Ps(highest_index);
    I_final = Is(highest_index);
    Dout_final = Douts(highest_index);
    Din_final  = Dins(highest_index);
else
    % disp("Interpolate!")
    P_final     = interp1(Zs,Ps,Zq,'spline');
    I_final     = interp1(Zs,Is,Zq,'spline');
    Dout_final  = interp1(Zs,Douts,Zq,'spline');
    Din_final   = interp1(Zs,Dins,Zq,'spline');
end



% Choose between "inner" and "outer" D gains
dz_mm = du * 1000;

if abs(dz_mm) <= du_inner_threshold
    % disp("Within inner threshold")
    D_final = Din_final;
elseif abs(dz_mm) >= du_outer_threshold
    % disp("Beyond outer threshold")
    D_final = Dout_final;
else
    % disp("In between; interpolate!")
    D_final = ( Dout_final- Din_final)*(abs(dz_mm) - du_inner_threshold)/(du_outer_threshold - du_inner_threshold) +  Din_final;
end


% Apply overrides (if any)
if ~isnan(P_override)
    P_final = P_override;
end
if ~isnan(I_override)
    I_final = I_override;
end
if ~isnan(D_override)
    D_final = D_override;
end
PID_out = [P_final, I_final, D_final];

== matlab function Z_3Dctrl/get_plant_input/Z_1dctrl/PID-Y/PID Gain scheduler/PID selector ==
  data: Ud input; du input; PIDDu_save input; du_inner_threshold input; du_outer_threshold input; PID_out output; P_override input; I_override input; D_override input
function PID_out = fcn(Ud,du,PIDDu_save,du_inner_threshold, du_outer_threshold, P_override,I_override,D_override)
% Interpolates for PID gains based on target Ud, using PID gains that were
% manually tuned at various target "Z" heights (with D gain being split into
% "near target height" and "far from target height" values, to allow for
% strong D contribution without risking destabilization near convergence).
% The "D" gain is then chosen between these aforementioned values based on
% how near/far the magnet is to Zd.

% Read recorded PID gains
Zq = Ud;

Ps = PIDDu_save(:,1);
Is = PIDDu_save(:,2);
Douts = PIDDu_save(:,3);
Dins = PIDDu_save(:,4);
Zs = PIDDu_save(:,5);
[~,lowest_index] = min(Zs);
[~,highest_index] = max(Zs);


% Interpolate if necessary!
if Ud <= Zs(lowest_index)
    % disp("Below 2mm!")
    P_final = Ps(lowest_index);
    I_final = Is(lowest_index);
    Dout_final = Douts(lowest_index);
    Din_final  = Dins(lowest_index);
elseif Ud >= Zs(highest_index)
    % disp("Above 5mm!")
    P_final = Ps(highest_index);
    I_final = Is(highest_index);
    Dout_final = Douts(highest_index);
    Din_final  = Dins(highest_index);
else
    % disp("Interpolate!")
    P_final     = interp1(Zs,Ps,Zq,'spline');
    I_final     = interp1(Zs,Is,Zq,'spline');
    Dout_final  = interp1(Zs,Douts,Zq,'spline');
    Din_final   = interp1(Zs,Dins,Zq,'spline');
end



% Choose between "inner" and "outer" D gains
dz_mm = du * 1000;

if abs(dz_mm) <= du_inner_threshold
    % disp("Within inner threshold")
    D_final = Din_final;
elseif abs(dz_mm) >= du_outer_threshold
    % disp("Beyond outer threshold")
    D_final = Dout_final;
else
    % disp("In between; interpolate!")
    D_final = ( Dout_final- Din_final)*(abs(dz_mm) - du_inner_threshold)/(du_outer_threshold - du_inner_threshold) +  Din_final;
end


% Apply overrides (if any)
if ~isnan(P_override)
    P_final = P_override;
end
if ~isnan(I_override)
    I_final = I_override;
end
if ~isnan(D_override)
    D_final = D_override;
end
PID_out = [P_final, I_final, D_final];

== matlab function Z_3Dctrl/Input parameters/Preset override ==
  data: XYZ_desired input; XYZ_desired_selection output; XYZ_preset_01 input; XYZ_preset_02 input; toggle input
function XYZ_desired_selection  = preset_override(XYZ_desired,XYZ_preset_01,XYZ_preset_02,toggle)
% Chooses between distinct XYZ_desired positions (default), or can toggle
% between that mode and preset XYZ_desired positions using parameter
% `toggle`.

% switch toggle
%     case 0
%         % Default mode
%         XYZ_desired_selection = XYZ_desired;
%     case 1
%         % Preset 01
%         XYZ_desired_selection = XYZ_preset_01;
%     case 2
%         % Preset 02
%         XYZ_desired_selection = XYZ_preset_02;
%     otherwise 
%         % Invalid; revert to default mode
%         XYZ_desired_selection = XYZ_desired;

if toggle >= 0 && toggle < 1
    % Default mode or Preset 01
    XYZ_desired_selection = XYZ_desired*(1-toggle) + XYZ_preset_01*(toggle);
elseif toggle >= 1 && toggle < 2
    % Preset 01
    toggle = toggle - 1;
    XYZ_desired_selection = XYZ_preset_01*(1-toggle) + XYZ_preset_02*(toggle);
elseif toggle >= 2 && toggle < 2.1
    % Preset 02 (no additional toggles implemented yet)
    toggle = toggle - 2;
    XYZ_desired_selection = XYZ_preset_02*(1-toggle) + XYZ_preset_02*(toggle);
else
    % Invalid; revert to default mode
    XYZ_desired_selection = XYZ_desired;
end
